simulink model "loading_simulation"  (R2015a)
settings: Solver=ode45  StartTime=0.0  StopTime=20  RelTol=1e-3
libraries: powerlib x3
settings Model: Creator=Lenovo  LastModifiedBy=Lenovo

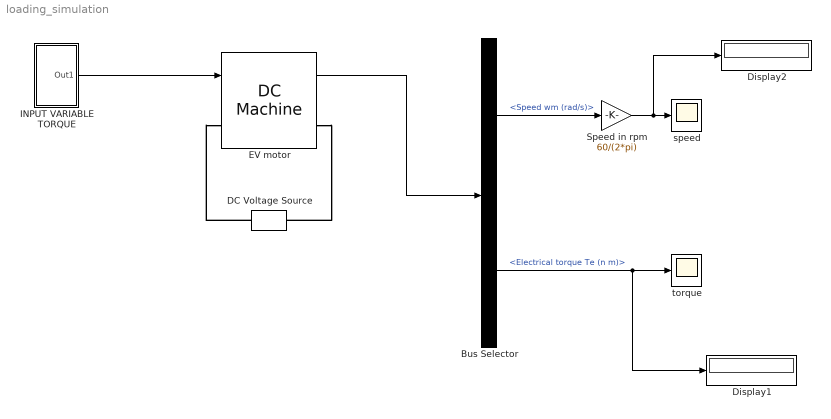
== system loading_simulation ==
  Bus Selector : BusSelector  OutputSignals=Speed wm (rad/s),Electrical torque Te (n m)
  DC Voltage Source : powerlib/Electrical Sources/DC Voltage Source  Amplitude=48  Measurements=None
  Display1 : Display
  Display2 : Display
  EV motor : powerlib/Machines/DC Machine  PresetModel=No  MechanicalLoad=Torque TL  FieldType=Permanent magnet  ShowDetailedParameters=on  MeasurementBus=off  RLa="[ 0.6  0.012]"  RLf="[ 240  120]"  Laf=1.8  MachineConstant=Torque constant (N.m/A)  Ke=1.8  Kt=1.8  J=1  Bm=0  Tf=0  w0=1  Ifinit=1  TsPowergui=0  TsBlock=-1
  INPUT VARIABLE TORQUE : Subsystem
  "Speed in rpm " : Gain  Gain=60/(2*pi)
  "speed " : Scope
  "torque " : Scope
      settings: SaveName=ScopeData2
  wires:
  Bus Selector/2 -> Display1/1, "torque "/1  "<Electrical torque Te (n m)>"
  Bus Selector/1 -> "Speed in rpm "/1  "<Speed wm (rad/s)>"
  "Speed in rpm "/1 -> Display2/1, "speed "/1
  EV motor/1 -> Bus Selector/1
  INPUT VARIABLE TORQUE/1(Out1) -> EV motor/1
  connections:
  DC Voltage Source/RConn1 -- EV motor/LConn1
  EV motor/RConn1 -- DC Voltage Source/LConn1

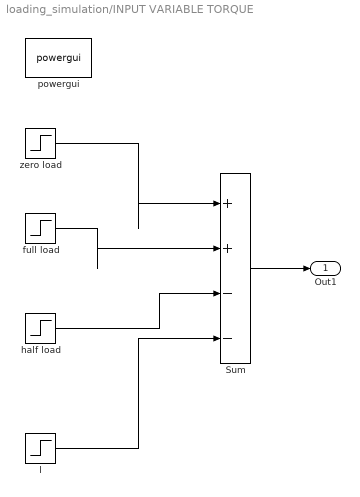
== system loading_simulation/INPUT VARIABLE TORQUE ==
  Sum : Sum  Inputs=|++--
  full load : Step  Time=5  After=28.8  SampleTime=0
  "half load " : Step  Time=10  After=14.4  SampleTime=0
  l : Step  Time=12  After=6  SampleTime=0
  powergui : powerlib/powergui  Priority=1  SimulationMode=Continuous  SolverType=Tustin/Backward Euler (TBE)  SampleTime=50e-6  frequency=60  SPID=off  DisableSnubberDevices=off  DisableRonSwitches=off  DisableVfSwitches=off  SwTol=0  DisplayEquations=off  Interpol=off  methode=off  Ts=100  FunctionMessages=off  echomessages=off  HookPort=off  EnableUseOfTLC=off  x0status=blocks  frequencyindice=0  Pbase=100e6  ErrMax=1e-4  Iterations=50  UnitsV=kV  UnitsW=MW  buscounter=0  RestoreLinks=warning  ResistiveCurrentMeasurement=off  Frange=[0:2:500]  Ylog=off  Xlog=on  ShowGrid=off  save=off  variable=ZData  structure=0  ZoomFFT=off  StartTime=0.0  cycles=1  DisplayStyle=1  fundamental=60  FreqAxis=off  MaxFrequency=1000  frequencyindicesteady=1  RmsSteady=1  display=off
  zero load : Step  Time=0  After=0  SampleTime=0
  Out1 : Outport
  wires:
  full load/1 -> Sum/2
  l/1 -> Sum/4
  "half load "/1 -> Sum/3
  zero load/1 -> Sum/1
  Sum/1 -> Out1/1
